simulink model "Regelaar"  (R2018b)
settings: Solver=FixedStepAuto  StartTime=0.0  StopTime=10  RelTol=1e-3
undefined symbols (not defined in the file or in its folder): A, B, DiscIntNeverNeededParam, Kdi, Tsc
libraries: simulink x2, pePwmGenerator x1, dspswit3 x1, dspsigops x1
settings Model: Creator=Roberto  LastModifiedBy=Roberto

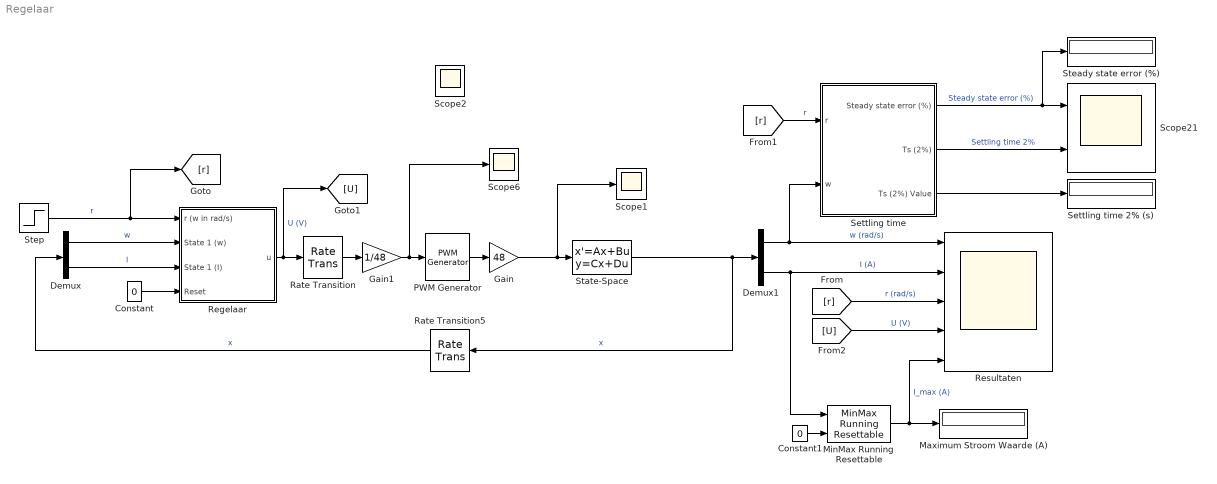
== system Regelaar ==
  Constant : Constant  Value=0
  Constant1 : Constant  Value=0
  Demux : Demux  Outputs=2
  Demux1 : Demux  Outputs=2
  Gain : Gain  Gain=48
  Gain1 : Gain  Gain=1/48
  Maximum Stroom Waarde (A) : Display
  MinMax Running Resettable : simulink/Math Operations/MinMax Running Resettable  Function=max  vinit=0.0
  PWM Generator : pePwmGenerator/PWM Generator  CarrCount=Up  Tper=1/20000  Ts=1e-6
  Rate Transition : RateTransition  OutPortSampleTime=1e-6
  Rate Transition5 : RateTransition  OutPortSampleTime=Tsc
  Regelaar : Subsystem
  Resultaten : Scope  NumInputPorts=5
  Scope1 : Scope
  Scope2 : Scope
  Scope21 : Scope  NumInputPorts=2
  Scope6 : Scope
  Settling time : Subsystem
  Settling time 2% (s) : Display
  State-Space : StateSpace  A=A  B=B  C=eye(2)  D=[0; 0]  InitialCondition=0
  Steady state error (%) : Display
  Step : Step  After=17  SampleTime=Tsc
  wires:
  Demux/1 -> Regelaar/2(State 1 (w))  "w"
  Demux/2 -> Regelaar/3(State 1 (I))  "I"
  State-Space/1 -> Rate Transition5/1, Demux1/1  "x"
  Constant/1 -> Regelaar/4(Reset)
  Step/1 -> [r], Regelaar/1(r (w in rad/s))  "r"
  Regelaar/1(u) -> [U], Rate Transition/1  "U (V)"
  Settling time/1(Steady state error (%)) -> Steady state error (%)/1, Scope21/1  "Steady state error (%)"
  Settling time/2(Ts (2%)) -> Scope21/2  "Settling time 2%"
  Demux1/1 -> Settling time/2(w), Resultaten/1  "w (rad/s)"
  Demux1/2 -> MinMax Running Resettable/1, Resultaten/2  "I (A)"
  [r] -> Resultaten/3  "r (rad/s)"
  [r] -> Settling time/1(r)  "r"
  Settling time/3(Ts (2%) Value) -> Settling time 2% (s)/1
  MinMax Running Resettable/1 -> Resultaten/5, Maximum Stroom Waarde (A)/1  "I_max (A)"
  Constant1/1 -> MinMax Running Resettable/2
  PWM Generator/1 -> Gain/1
  Gain1/1 -> Scope6/1, PWM Generator/1
  Rate Transition/1 -> Gain1/1
  Gain/1 -> State-Space/1, Scope1/1
  Rate Transition5/1 -> Demux/1  "x"
  [U] -> Resultaten/4  "U (V)"

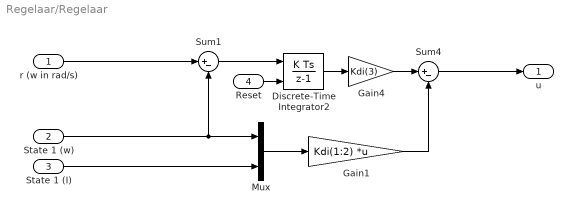
== system Regelaar/Regelaar ==
  r (w in rad/s) : Inport
  State 1 (w) : Inport  Port=2
  State 1 (I) : Inport  Port=3
  Reset : Inport  Port=4
  Discrete-Time Integrator2 : DiscreteIntegrator  gainval=1  ExternalReset=rising  SampleTime=Tsc  ICPrevOutput=DiscIntNeverNeededParam  ICPrevScaledInput=DiscIntNeverNeededParam
  Gain1 : Gain  Gain=Kdi(1:2)  Multiplication=Matrix(K*u)
  Gain4 : Gain  Gain=Kdi(3)
  Mux : Mux  Inputs=2
  Sum1 : Sum  Inputs=|+-
  Sum4 : Sum  Inputs=|+-
  u : Outport
  wires:
  r (w in rad/s)/1 -> Sum1/1
  State 1 (I)/1 -> Mux/2
  Mux/1 -> Gain1/1
  Gain1/1 -> Sum4/2
  Gain4/1 -> Sum4/1
  Sum4/1 -> u/1
  State 1 (w)/1 -> Mux/1, Sum1/2
  Sum1/1 -> Discrete-Time Integrator2/1
  Discrete-Time Integrator2/1 -> Gain4/1
  Reset/1 -> Discrete-Time Integrator2/2

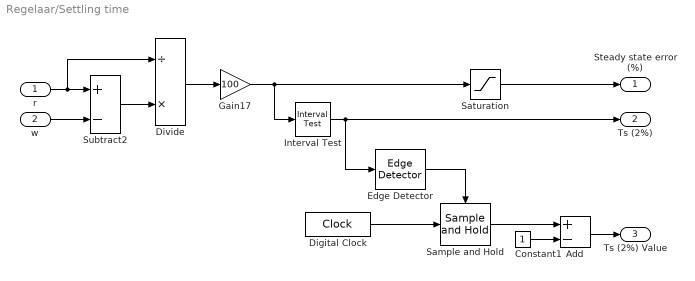
== system Regelaar/Settling time ==
  r : Inport
  w : Inport  Port=2
  Add : Sum  Inputs=+-
  Constant1 : Constant
  Digital Clock : DigitalClock  SampleTime=Tsc
  Divide : Product  Inputs=/*
  Edge Detector : dspswit3/Edge Detector  InputProcessing=Columns as channels (frame based)
      settings: SourceProductName=DSP System Toolbox  SourceProductBaseCode=DS
  Gain17 : Gain  Gain=100
  Interval Test : simulink/Logic and Bit Operations/Interval Test  IntervalClosedRight=on  uplimit=2  IntervalClosedLeft=on  lowlimit=-2  OutDataTypeStr=boolean
  Sample and Hold : dspsigops/Sample and Hold  trig=Rising edge  initCond=0  latchinput=off
  Saturation : Saturate  UpperLimit=3  LowerLimit=-3
  Subtract2 : Sum  Inputs=+-
  Steady state error (%) : Outport
  Ts (2%) : Outport  Port=2
  Ts (2%) Value : Outport  Port=3
  wires:
  Divide/1 -> Gain17/1
  r/1 -> Subtract2/1, Divide/1
  Gain17/1 -> Saturation/1, Interval Test/1
  Subtract2/1 -> Divide/2
  w/1 -> Subtract2/2
  Edge Detector/1 -> Sample and Hold/Trigger
  Sample and Hold/1 -> Add/1
  Interval Test/1 -> Ts (2%)/1, Edge Detector/1
  Digital Clock/1 -> Sample and Hold/1
  Constant1/1 -> Add/2
  Add/1 -> Ts (2%) Value/1
  Saturation/1 -> Steady state error (%)/1
